simulink model "Half_Adder"  (R2020a)
settings: Solver=VariableStepAuto  StartTime=0.0  StopTime=10.0  RelTol=1e-3
settings Model: Creator=ashwin  LastModifiedBy=ashwin

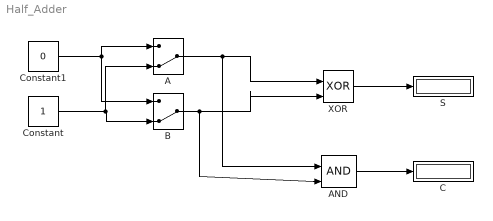
== system Half_Adder ==
  A : ManualSwitch  CurrentSetting=0
  AND : Logic  IconShape=distinctive  AllPortsSameDT=off  OutDataTypeStr=boolean
  B : ManualSwitch  CurrentSetting=0
  C : Display
  Constant : Constant
  Constant1 : Constant  Value=0
  S : Display
  XOR : Logic  Operator=XOR  IconShape=distinctive  AllPortsSameDT=off  OutDataTypeStr=boolean
  wires:
  A/1 -> AND/1, XOR/1
  B/1 -> AND/2, XOR/2
  Constant1/1 -> A/1, B/1
  Constant/1 -> A/2, B/2
  AND/1 -> C/1
  XOR/1 -> S/1
